simulink model "power_battery_powersim"  (Simulink 8.9)
settings: Solver=ode23tb  StartTime=0.0  StopTime=3600  MaxStep=0.1  RelTol=1e-4  EnableMultiTasking=on
undefined symbols (not defined in the file): Acid, Lead
libraries: powerlib x3, electricdrivelib x1
Description:
  | Copyright 2008-2017 The MathWorks, Inc.
settings Model: SuppressorTable=22 serialization::archive 11 0 6 0 0 0 0 0  Creator=MathWorks  LastModifiedBy=judithlopez
settings OptimizationCC: ExpressionDepthLimit=2147483647  InitFltsAndDblsToZero=on
settings DebuggingCC: SignalResolutionControl=TryResolveAllWithWarning  SolverPrmCheckMsg=warning  AllowSymbolicDim=off

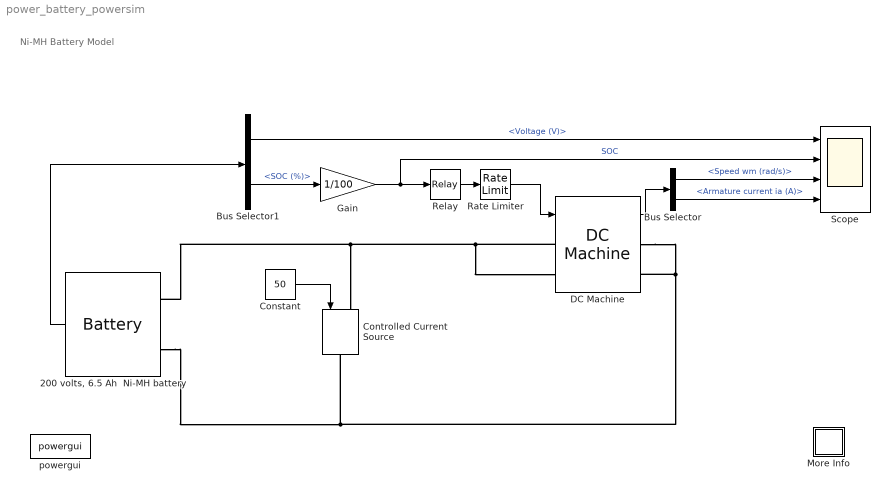
== system power_battery_powersim ==
  note: Ni-MH Battery Model
  "200 volts, 6.5 Ah  Ni-MH battery " : electricdrivelib/Extra Sources/Battery  BatType=Lead-Acid  ShowTempParam=on  ThermalPreset="11.1V  6600mAh  (LiCoO2)"  ShowAgeParam=off  NomV=12  NomQ=1.2  SOC=100  Batt_Tr=30  PresetModel=on  MaxQ=1.25  MinV=9  FullV=13.0658  Dis_rate=0.24  R=0.1  Normal_OP=0.37233  expZone="[12.2171        0.004]"  current=50  Units=Ampere-hour  Tci=20  NomT=21  T2=-10  MaxQ2=6.48  FullV2=11.28  Normal_OP2=9.37  expZone2="[11         0.07]"  Rca=1.2  ti=1000  Dp=0  Neq0=0  Tsim=1e6  Ta1=25  Qeol=5.4*0.9  Reol=0.013333*1.2  Char_age=[2.3478, 3]  Dis_age=[2.3478, 10]  N1=1500  N2=10500  N3=1000  N4=1400  Ta2=45  N5=950
  Bus Selector : BusSelector  OutputSignals=Speed wm (rad/s),Armature current ia (A)
  Bus Selector1 : BusSelector  OutputSignals=Voltage (V),SOC (%)
  Constant : Constant  Value=50
  Controlled Current Source : powerlib/Electrical Sources/Controlled Current Source  Initialize=on  Source_Type=AC  Amplitude=0  Phase=0  Frequency=0  Measurements=None
  DC Machine : powerlib/Machines/DC Machine  PresetModel=No  MechanicalLoad=Torque TL  FieldType=Wound  ShowDetailedParameters=on  MeasurementBus=off  RLa=[0.4832 0.006763]  RLf=[84.91 13.39]  Laf=0.7096  MachineConstant=Torque constant (N.m/A)  Ke=1.8  Kt=1.8  J=0.2053  Bm=0.007032  Tf=0  w0=0  Ifinit=0  TsPowergui=0  TsBlock=-1
  Gain : Gain  Gain=1/100
  More Info : Subsystem
      settings: OpenFcn=showdemo(bdroot(gcb))
      mask Display: disp('?')
  Rate Limiter : RateLimiter  RisingSlewLimit=100  FallingSlewLimit=-100
  Relay : Relay  OnSwitchValue=0.8  OffSwitchValue=0.4  OnOutputValue=0  OffOutputValue=-200
  Scope : Scope  NumInputPorts=4
  powergui : powerlib/powergui  SimulationMode=Continuous  SampleTime=0.001  frequency=60  Iterations=50  frequencyindice=0  Pbase=100e6  ErrMax=1e-4  UnitsV=kV  UnitsW=MW  buscounter=0  FunctionMessages=off  echomessages=off  EnableUseOfTLC=off  CurrentSourceSwitches=off  DisableSnubberDevices=off  DisableRonSwitches=off  DisableVfSwitches=off  DisplayEquations=off  SolverType=Tustin  Interpol=off  ExternalGateDelay=off  methode=off  Ts=0  x0status=blocks  SPID=off  SwTol=0  HookPort=off  RestoreLinks=warning  ResistiveCurrentMeasurement=off  Frange=[0:2:500]  Ylog=off  Xlog=on  ShowGrid=off  save=off  variable=ZData  structure=0  ZoomFFT=on  StartTime=0.0  cycles=1  DisplayStyle=1  fundamental=60  FreqAxis=off  MaxFrequency=1000  frequencyindicesteady=1  RmsSteady=1  display=off
  wires:
  DC Machine/1 -> Bus Selector/1
  Constant/1 -> Controlled Current Source/1
  Relay/1 -> Rate Limiter/1
  Bus Selector/1 -> Scope/3  "<Speed wm (rad/s)>"
  Bus Selector/2 -> Scope/4  "<Armature current ia (A)>"
  Rate Limiter/1 -> DC Machine/1
  "200 volts, 6.5 Ah  Ni-MH battery "/1 -> Bus Selector1/1
  Bus Selector1/2 -> Gain/1  "<SOC (%)>"
  Gain/1 -> Relay/1, Scope/2  "SOC"
  Bus Selector1/1 -> Scope/1  "<Voltage (V)>"
  connections:
  "200 volts, 6.5 Ah  Ni-MH battery "/LConn2 -- DC Machine/RConn1 -- DC Machine/RConn2 -- Controlled Current Source/RConn1
  "200 volts, 6.5 Ah  Ni-MH battery "/LConn1 -- DC Machine/LConn1 -- DC Machine/LConn2 -- Controlled Current Source/LConn1

== system power_battery_powersim/More Info ==
